simulink model "SimLTI"  (R2017a)
settings: Solver=FixedStepAuto  StartTime=0.0  StopTime=time(end)  FixedStep=.01  RelTol=1e-3  EnableMultiTasking=on
PostLoadFcn:
  | load LTI_data_2017-11-06_16-22.mat
  | load Trajectory_data_Cux_Visby.rtz2017-11-16_14-55.mat
undefined symbols (not defined in the file): Dr, Du, toMpS, toRad, toRPS
libraries: cstblocks x1
settings Model: Creator=c00rts11  LastModifiedBy=c00rts11
settings SolverCC: ZeroCrossAlgorithm=Adaptive

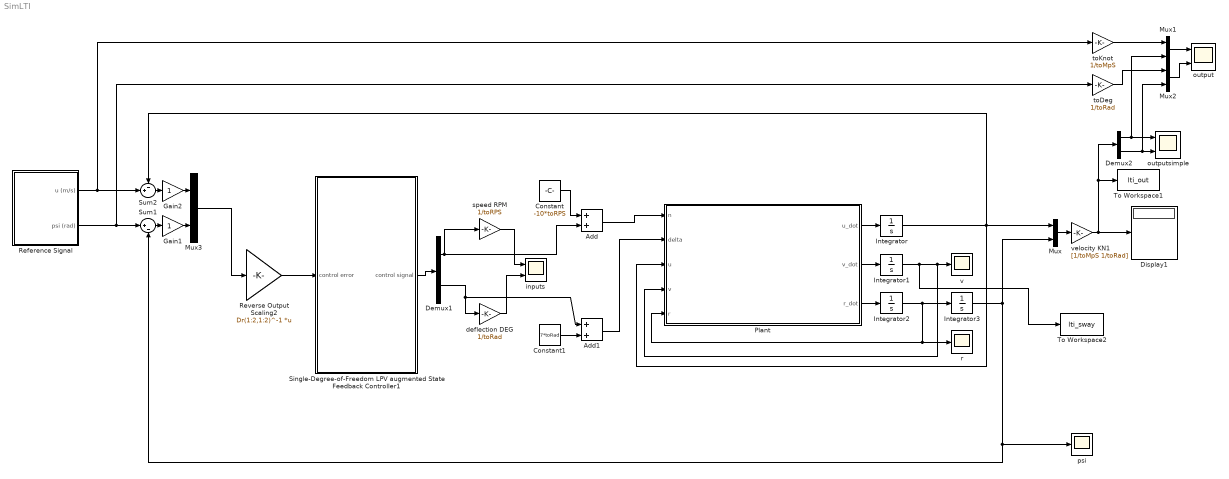
== system SimLTI ==
  Add : Sum
  Add1 : Sum
  Constant : Constant  Value=-10*toRPS
  Constant1 : Constant  Value=7*toRad
  Demux1 : Demux  Outputs=2
  Demux2 : Demux  Outputs=2
  Display1 : Display
  Gain1 : Gain
  Gain2 : Gain
  Integrator : Integrator  InitialCondition=.1*toMpS  UpperSaturationLimit=16*toMpS  LowerSaturationLimit=1e-1*toMpS
  Integrator1 : Integrator  UpperSaturationLimit=0*toMpS  LowerSaturationLimit=-0.001*toMpS
  Integrator2 : Integrator
  Integrator3 : Integrator  UpperSaturationLimit=180*toRad  LowerSaturationLimit=-180*toRad  WrapState=on  WrappedStateUpperValue=180*toRad  WrappedStateLowerValue=-180*toRad  IgnoreLimit=on
  Mux{,1..3} (4 alike) : Mux  Inputs=2
  Plant : MATLAB Function  TreatAsAtomicUnit=on
  Reference Signal : Subsystem
  Reverse Output Scaling2 : Gain  Gain=Dr(1:2,1:2)^-1  Multiplication=Matrix(K*u)
  Single-Degree-of-Freedom LPV augmented State Feedback Controller1 : Subsystem
  Sum1 : Sum  Inputs=|+-
  Sum2 : Sum  Inputs=-+|
  To Workspace1 : ToWorkspace  VariableName=lti_out  SaveFormat=Timeseries  SampleTime=-1
  To Workspace2 : ToWorkspace  VariableName=lti_sway  SaveFormat=Timeseries  SampleTime=-1
  deflection DEG : Gain  Gain=1/toRad
  inputs : Scope  NumInputPorts=2
  output : Scope  NumInputPorts=2
  outputsimple : Scope  NumInputPorts=2
  psi : Scope
  r : Scope
  speed RPM : Gain  Gain=1/toRPS
  toDeg : Gain  Gain=1/toRad
  toKnot : Gain  Gain=1/toMpS
  v : Scope
  velocity KN1 : Gain  Gain=[1/toMpS 1/toRad]
  wires:
  Plant/2(v_dot) -> Integrator1/1
  Plant/3(r_dot) -> Integrator2/1
  Mux/1 -> velocity KN1/1
  Plant/1(u_dot) -> Integrator/1
  Single-Degree-of-Freedom LPV augmented State Feedback Controller1/1(control signal) -> Demux1/1
  Reverse Output Scaling2/1 -> Single-Degree-of-Freedom LPV augmented State Feedback Controller1/1(control error)
  Integrator3/1 -> Mux/2, Sum1/2, psi/1
  Sum1/1 -> Gain1/1
  Gain1/1 -> Mux3/2
  speed RPM/1 -> inputs/1
  Demux1/1 -> Add/2, speed RPM/1
  Demux1/2 -> Add1/1, deflection DEG/1
  deflection DEG/1 -> inputs/2
  Mux3/1 -> Reverse Output Scaling2/1
  Integrator/1 -> Sum2/1, Mux/1, Plant/3(u)
  Sum2/1 -> Gain2/1
  Gain2/1 -> Mux3/1
  Integrator2/1 -> Integrator3/1, r/1, Plant/5(r)
  velocity KN1/1 -> To Workspace1/1, Demux2/1, Display1/1
  Integrator1/1 -> To Workspace2/1, Plant/4(v), v/1
  Mux2/1 -> output/2
  Mux1/1 -> output/1
  Demux2/2 -> Mux2/2, outputsimple/2
  Demux2/1 -> Mux1/2, outputsimple/1
  toDeg/1 -> Mux2/1
  Constant/1 -> Add/1
  Add/1 -> Plant/1(n)
  Constant1/1 -> Add1/2
  Add1/1 -> Plant/2(delta)
  Reference Signal/1(u (m/s)) -> toKnot/1, Sum2/2
  Reference Signal/2(psi (rad)) -> toDeg/1, Sum1/1
  toKnot/1 -> Mux1/1

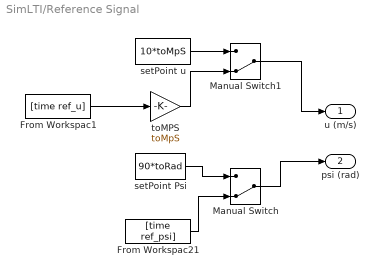
== system SimLTI/Reference Signal ==
  From Workspac1 : FromWorkspace  VariableName=[time ref_u]  SampleTime=0  Interpolate=off  OutputAfterFinalValue=Holding final value
  From Workspac21 : FromWorkspace  VariableName=[time ref_psi]  SampleTime=0  Interpolate=off  OutputAfterFinalValue=Holding final value
  Manual Switch : ManualSwitch  CurrentSetting=0
  Manual Switch1 : ManualSwitch  CurrentSetting=0
  setPoint Psi : Constant  Value=90*toRad
  setPoint u : Constant  Value=10*toMpS
  toMPS : Gain  Gain=toMpS
  u (m/s) : Outport
  psi (rad) : Outport  Port=2
  wires:
  From Workspac21/1 -> Manual Switch/2
  toMPS/1 -> Manual Switch1/2
  Manual Switch1/1 -> u (m/s)/1
  setPoint u/1 -> Manual Switch1/1
  setPoint Psi/1 -> Manual Switch/1
  Manual Switch/1 -> psi (rad)/1
  From Workspac1/1 -> toMPS/1

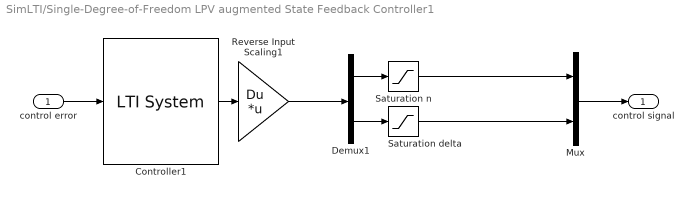
== system SimLTI/Single-Degree-of-Freedom LPV augmented State Feedback Controller1 ==
  control error : Inport
  Controller1 : cstblocks/LTI System  sys=K  IC=[]
  Demux1 : Demux  Outputs=2
  Mux : Mux  Inputs=2
  Reverse Input Scaling1 : Gain  Gain=Du  Multiplication=Matrix(K*u)
  Saturation delta : Saturate  UpperLimit=10*toRad  LowerLimit=-10*toRad
  Saturation n : Saturate  UpperLimit=80*toRPS  LowerLimit=-80*toRPS  LinearizeAsGain=off
  control signal : Outport
  wires:
  control error/1 -> Controller1/1
  Controller1/1 -> Reverse Input Scaling1/1
  Demux1/1 -> Saturation n/1
  Saturation delta/1 -> Mux/2
  Saturation n/1 -> Mux/1
  Reverse Input Scaling1/1 -> Demux1/1
  Demux1/2 -> Saturation delta/1
  Mux/1 -> control signal/1

== matlab function SimLTI/Plant ==
  data: n input; delta input; u input; u_dot output; v input; r input; v_dot output; r_dot output
function [u_dot,v_dot,r_dot] = fcn(n,delta,u,v,r)
% n = n/60;
% v = 0;
% r = 0;
if (u==0)
    u = 1e-1;
end
% Normalization variables
L   =  304.8;          % length of ship (m)
g   =  9.8;            % acceleration of gravity (m/s^2)

% Parameters, hydrodynamic derivatives and main dimensions
% delta_max  = 10;       % max rudder angle      (deg)
% Ddelta_max = 2.33;     % max rudder derivative (deg/s)
% n_max      = 80;       % max shaft velocity    (rpm)

t   =  0.22;
Tm  =  50;
T   =  18.46;

cun =  0.605;  
cnn =  38.2;

Tuu = -0.00695;
Tun = -0.00063;
Tnn =  0.0000354;

m11 =  1.050;          % 1 - Xudot
m22 =  2.020;          % 1 - Yvdot
m33 =  0.1232;         % kz^2 - Nrdot

d11 =  2.020;          % 1 + Xvr
d22 = -0.752;          % Yur - 1
d33 = -0.231;          % Nur - xG 

Xuuz   = -0.0061;   YT     =  0.04;   NT      = -0.02;
Xuu    = -0.0377;   Yvv    = -2.400;  Nvr     = -0.300;
Xvv    =  0.3;      Yuv    = -1.205;  Nuv     = -0.451;   
Xudotz = -0.05;     Yvdotz = -0.387;  Nrdotz  = -0.0045;
Xuuz   = -0.0061;   Yurz   =  0.182;  Nurz    = -0.047;
Xvrz   =  0.387;    Yvvz   = -1.5;    Nvrz    = -0.120;
Xccdd  = -0.093;    Yuvz   =  0;      Nuvz    = -0.241;
Xccbd  =  0.152;    Yccd   =  0.208;  Nccd    = -0.098;
Xvvzz  =  0.0125;   Yccbbd = -2.16;   Nccbbd  =  0.688;
                    Yccbbdz= -0.191;  Nccbbdz =  0.344;

z = T./(50 - T);

% Forces and moments
beta = v/u;
gT   = (1/L*Tuu*u^2 + Tun*u*n + L*Tnn*abs(n)*n);
% C = (cun*u*n + cnn*n^2)*sign(cun*u*n + cnn*n^2);
C = (cun*u*n + cnn*n^2);

gX   = 1/L*(Xuu*u^2 + L*d11*v*r + Xvv*v^2 + Xccdd*C*delta^2 ...
     + Xccbd*C*beta*delta + L*gT*(1-t) + Xuuz*u^2*z ...
     + L*Xvrz*v*r*z + Xvvzz*v^2*z^2);

gY   = 1/L*(Yuv*u*v + Yvv*abs(v)*v + Yccd*C*delta + L*d22*u*r ...
     + Yccbbd*C*abs(beta)*beta*abs(delta) + YT*gT*L ...
     + L*Yurz*u*r*z + Yuvz*u*v*z + Yvvz*abs(v)*v*z  ...
     + Yccbbdz*C*abs(beta)*beta*abs(delta)*z);     

gLN  = Nuv*u*v + L*Nvr*abs(v)*r + Nccd*C*delta +L*d33*u*r ...
     + Nccbbd*C*abs(beta)*beta*abs(delta) + L*NT*gT ...
     + L*Nurz*u*r*z + Nuvz*u*v*z + L*Nvrz*abs(v)*r*z ...
     + Nccbbdz*C*abs(beta)*beta*abs(delta)*z;
 
%  c    = sqrt(cun*u*n + cnn*n^2);
% 
% gX   = 1/L*(Xuu*u^2 + L*d11*v*r + Xvv*v^2 + Xccdd*abs(c)*c*delta^2 ...
%      + Xccbd*abs(c)*c*beta*delta + L*gT*(1-t) + Xuuz*u^2*z ...
%      + L*Xvrz*v*r*z + Xvvzz*v^2*z^2);
% 
% gY   = 1/L*(Yuv*u*v + Yvv*abs(v)*v + Yccd*abs(c)*c*delta + L*d22*u*r ...
%      + Yccbbd*abs(c)*c*abs(beta)*beta*abs(delta) + YT*gT*L ...
%      + L*Yurz*u*r*z + Yuvz*u*v*z + Yvvz*abs(v)*v*z  ...
%      + Yccbbdz*abs(c)*c*abs(beta)*beta*abs(delta)*z);     
% 
% gLN  = Nuv*u*v + L*Nvr*abs(v)*r + Nccd*abs(c)*c*delta +L*d33*u*r ...
%      + Nccbbd*abs(c)*c*abs(beta)*beta*abs(delta) + L*NT*gT ...
%      + L*Nurz*u*r*z + Nuvz*u*v*z + L*Nvrz*abs(v)*r*z ...
%      + Nccbbdz*abs(c)*c*abs(beta)*beta*abs(delta)*z;

m11 = (m11 - Xudotz*z);
m22 = (m22 - Yvdotz*z);
m33 = (m33 - Nrdotz*z);

% Dimensional state derivative
u_dot = gX/m11;
v_dot = gY/m22;
r_dot = gLN/(L^2*m33);
